simulink model "s_bb01_pos_outer_loop"  (R2021b)
settings: Solver=ode4  StartTime=0.0  StopTime=25  FixedStep=0.002  RelTol=1e-3  AbsTol=1e-6  EnableMultiTasking=on
values from neighbouring files (symbols this model uses):
  K_bb = m_b * g * r_arm / L_beam * r_b^2 / ( m_b * r_b^2 + J_b )    [d_bb01_model_param.m]    (also in setup_srv02_exp04_bb01.m = 0)
  Kc = wn^2 / (Tp*K_bb*z*wf)    [d_bb01_pd.m]    (also in setup_srv02_exp04_bb01.m = 0)
  THETA_MAX = 56.0 * K_D2R    [config_bb01.m]
  THETA_MIN = - 56.0 * K_D2R    [config_bb01.m]
  z = wn*wf/(-wn+wf*wn*Tp+2*wf*zeta)    [d_bb01_pd.m]    (also in setup_srv02_exp04_bb01.m = 1)
libraries: simulink x3, simulink_extras x1
settings Model: ExtModeTrigDuration=10000  Creator=MLevis  LastModifiedBy=Dell
settings SolverCC: AutoScaleAbsTol=off  AlgebraicLoopSolver=TrustRegion  PositivePriorityOrder=on
settings DataIOCC: SaveFormat=Array  SignalLoggingSaveFormat=ModelDataLogs  ReturnWorkspaceOutputs=off
settings OptimizationCC: BlockReduction=off  BooleanDataType=off  OptimizeBlockIOStorage=off  BufferReuse=off  ExpressionFolding=off  ExpressionDepthLimit=2147483647  LocalBlockOutputs=off  InitFltsAndDblsToZero=on
settings DebuggingCC: SaveWithParameterizedLinksMsg=none  UnderspecifiedInitializationDetection=Classic  MergeDetectMultiDrivingBlocksExec=none  SignalResolutionControl=TryResolveAllWithWarning  MultiTaskDSMMsg=warning  MultiTaskCondExecSysMsg=none  FcnCallInpInsideContextMsg=warning  StateNameClashWarn=warning  SFUnexpectedBacktrackingDiag=warning  SFNoUnconditionalDefaultTransitionDiag=warning  SFExecutionAtInitializationDiag=none  SFMachineParentedDataDiag=warning  ArithmeticOperatorsInVariantConditions=warning
settings HardwareCC: ProdBitPerPointer=32  ProdBitPerSizeT=32  ProdBitPerPtrDiffT=32  ProdWordSize=32  ProdHWDeviceType=Intel->x86-32 (Windows32)
settings ModelReferenceCC: PropagateSignalLabelsOutOfModel=off
settings RTWCC: Description=QUARC Win32 Target Using Toolchain  SystemTargetFile=quarc_windows.tlc  TemplateMakefile=quarc_default_tmf  Toolchain=QUARC windows | nmake (64-bit Windows)  BuildConfiguration=Faster Runs
settings CodeAppCC: StateflowObjectComments=on
settings STFCustomTargetCC: ConcurrentExecutionCompliant=on  UseToolchainInfoCompliant=on  SystemTargetFile=quarc_windows.tlc
settings GRTTargetCC: TargetLangStandard=C89/C90 (ANSI)  ParMdlRefBuildCompliant=off  CompOptLevelCompliant=off  CombineOutputUpdateFcns=off  MatFileLogging=off  CPPClassGenCompliant=off  GRTInterface=on  ExtMode=on  ExtModeMexFile=quarc_comm
settings ConfigComp: CovMetricSettings=dw  CovSaveCumulativeToWorkspaceVar=on  CovSaveSingleToWorkspaceVar=on

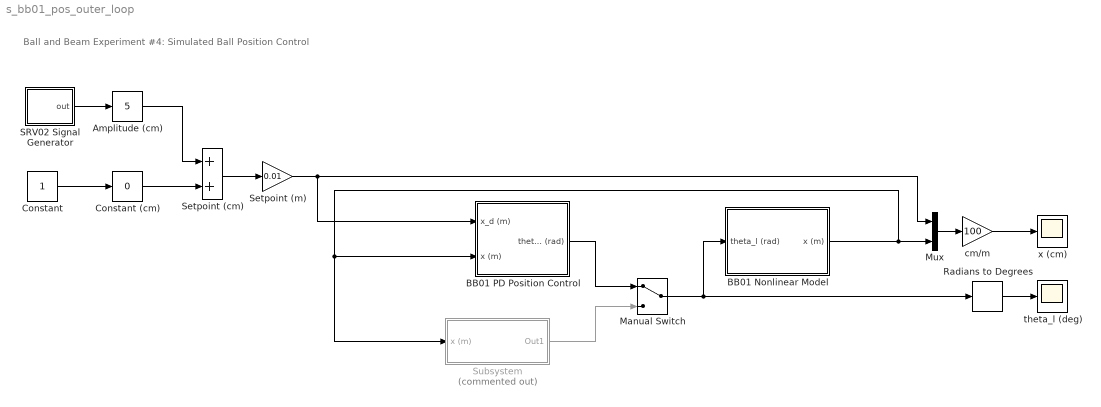
== system s_bb01_pos_outer_loop ==
  note: Ball and Beam Experiment #4: Simulated Ball Position Control
  Amplitude (cm) : simulink/Math Operations/Slider Gain  gain=5  low=-10  high=10
  BB01 Nonlinear Model : Subsystem
  BB01 PD Position Control : Subsystem
  "Constant " : Constant
  Constant (cm) : simulink/Math Operations/Slider Gain  gain=0  low=-20  high=20
  Manual Switch : ManualSwitch
  Mux : Mux  Inputs=2
  Radians to Degrees : simulink_extras/Transformations/Radians to Degrees
  SRV02 Signal Generator : Subsystem  mask(QET Signal Generator){sig_type=square, a=1, f=0.05}
      mask prompts: sig_type "Signal Type"; a "Amplitude"; f "Frequency (Hz)"
      mask help: Generates a square, triangular, or sinusoidal waveform of a specified amplitude and frequency.
      mask Help: Choose the type of signal to be generated from the drop-down "Signal Type" box. Enter the amplitude and the frequency desired for the signal. Note: frequency is in Hertz.
      mask TypeOptions sig_type: square | triangle | sine
      mask Display: plot([0 1 1 2 2 3 4 5 6], [-1 -1 1 1 -1 -1 1 -1 -1])
  Setpoint (cm) : Sum
  Setpoint (m) : Gain  Gain=0.01
  Subsystem : Subsystem  Commented=on
  cm/m : Gain  Gain=100
  theta_l (deg) : Scope
  x (cm) : Scope
  wires:
  Mux/1 -> cm/m/1
  Manual Switch/1 -> Radians to Degrees/1, BB01 Nonlinear Model/1(theta_l (rad))
  SRV02 Signal Generator/1(out) -> Amplitude (cm)/1
  Constant (cm)/1 -> Setpoint (cm)/2
  "Constant "/1 -> Constant (cm)/1
  Amplitude (cm)/1 -> Setpoint (cm)/1
  Setpoint (cm)/1 -> Setpoint (m)/1
  Setpoint (m)/1 -> Mux/1, BB01 PD Position Control/1(x_d (m))
  Radians to Degrees/1 -> theta_l (deg)/1
  cm/m/1 -> x (cm)/1
  BB01 Nonlinear Model/1(x (m)) -> Mux/2, Subsystem/1(x (m)), BB01 PD Position Control/2(x (m))
  Subsystem/1(Out1) -> Manual Switch/2
  BB01 PD Position Control/1(theta_d (rad)) -> Manual Switch/1

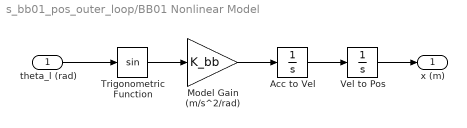
== system s_bb01_pos_outer_loop/BB01 Nonlinear Model ==
  theta_l (rad) : Inport
  Acc to Vel : Integrator
  Model Gain (m/s^2/rad) : Gain  Gain=K_bb
  Trigonometric Function : Trigonometry
  Vel to Pos : Integrator
  x (m) : Outport
  wires:
  Vel to Pos/1 -> x (m)/1
  Model Gain (m/s^2/rad)/1 -> Acc to Vel/1
  Acc to Vel/1 -> Vel to Pos/1
  theta_l (rad)/1 -> Trigonometric Function/1
  Trigonometric Function/1 -> Model Gain (m/s^2/rad)/1

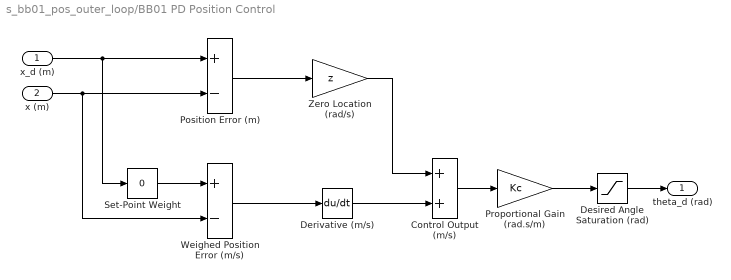
== system s_bb01_pos_outer_loop/BB01 PD Position Control ==
  x_d (m) : Inport
  x (m) : Inport  Port=2
  Control Output (m/s) : Sum
  Derivative (m/s) : Derivative
  Desired Angle Saturation (rad) : Saturate  UpperLimit=THETA_MAX  LowerLimit=THETA_MIN
  Position Error (m) : Sum  Inputs=+-
  Proportional Gain (rad.s/m) : Gain  Gain=Kc
  Set-Point Weight : simulink/Math Operations/Slider Gain  gain=0  low=0  high=1
  Weighed Position Error (m/s) : Sum  Inputs=+-
  Zero Location (rad/s) : Gain  Gain=z
  theta_d (rad) : Outport
  wires:
  Desired Angle Saturation (rad)/1 -> theta_d (rad)/1
  x (m)/1 -> Position Error (m)/2, Weighed Position Error (m/s)/2
  x_d (m)/1 -> Position Error (m)/1, Set-Point Weight/1
  Control Output (m/s)/1 -> Proportional Gain (rad.s/m)/1
  Proportional Gain (rad.s/m)/1 -> Desired Angle Saturation (rad)/1
  Set-Point Weight/1 -> Weighed Position Error (m/s)/1
  Weighed Position Error (m/s)/1 -> Derivative (m/s)/1
  Position Error (m)/1 -> Zero Location (rad/s)/1
  Zero Location (rad/s)/1 -> Control Output (m/s)/1
  Derivative (m/s)/1 -> Control Output (m/s)/2

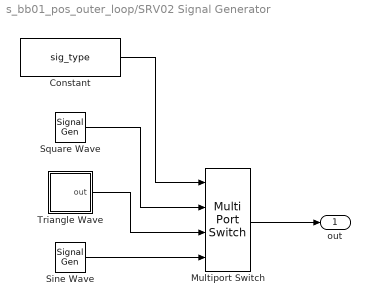
== system s_bb01_pos_outer_loop/SRV02 Signal Generator ==
  Constant : Constant  Value=sig_type
  Multiport Switch : MultiPortSwitch
  Sine Wave : SignalGenerator  Amplitude=a  Frequency=f
  Square Wave : SignalGenerator  WaveForm=square  Amplitude=a  Frequency=f
  Triangle Wave : Subsystem
  out : Outport
  wires:
  Square Wave/1 -> Multiport Switch/2
  Triangle Wave/1(out) -> Multiport Switch/3
  Sine Wave/1 -> Multiport Switch/4
  Multiport Switch/1 -> out/1
  Constant/1 -> Multiport Switch/1

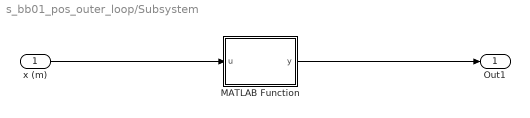
== system s_bb01_pos_outer_loop/Subsystem ==
  x (m) : Inport
  MATLAB Function : MATLAB Function  TreatAsAtomicUnit=on
  Out1 : Outport
  wires:
  x (m)/1 -> MATLAB Function/1(u)
  MATLAB Function/1(y) -> Out1/1

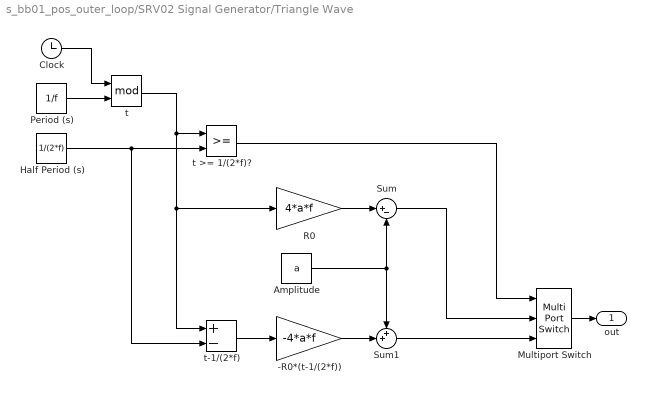
== system s_bb01_pos_outer_loop/SRV02 Signal Generator/Triangle Wave ==
  -R0*(t-1/(2*f)) : Gain  Gain=-4*a*f
  Amplitude : Constant  Value=a
  Clock : Clock
  Half Period (s) : Constant  Value=1/(2*f)
  Multiport Switch : MultiPortSwitch  DataPortOrder=Zero-based contiguous  Inputs=2  zeroidx=on
  Period (s) : Constant  Value=1/f
  R0 : Gain  Gain=4*a*f
  Sum : Sum  Inputs=|+-
  Sum1 : Sum  Inputs=++|
  t : Math  Operator=mod  SignedPower=on  SaturateOnIntegerOverflow=on
  t >= 1/(2*f)? : RelationalOperator  OutDataTypeStr=boolean  RndMeth=Nearest
  t-1/(2*f) : Sum  Inputs=+-
  out : Outport
  wires:
  Sum1/1 -> Multiport Switch/3
  Sum/1 -> Multiport Switch/2
  t >= 1/(2*f)?/1 -> Multiport Switch/1
  -R0*(t-1/(2*f))/1 -> Sum1/2
  Amplitude/1 -> Sum1/1, Sum/2
  R0/1 -> Sum/1
  t-1/(2*f)/1 -> -R0*(t-1/(2*f))/1
  Half Period (s)/1 -> t-1/(2*f)/2, t >= 1/(2*f)?/2
  t/1 -> t-1/(2*f)/1, R0/1, t >= 1/(2*f)?/1
  Period (s)/1 -> t/2
  Clock/1 -> t/1
  Multiport Switch/1 -> out/1

== matlab function s_bb01_pos_outer_loop/Subsystem/MATLAB Function ==
  data: u input; y output
function y = fcn(u)

A = [0,1:0,0];
B = [0;0.418];
C = [1,0];
D = 0;
sys = ss(A,B,C,D);

Q = eye(2);
R = 1;

[K,S,e] = lqr(sys, Q, R);

y = -K(1) * u;
